simulink model "Test_iowahills_IIR"  (R2017b)
settings: Solver=FixedStepDiscrete  StartTime=0.0  StopTime=0.01  FixedStep=1/245.76e6  RelTol=1e-3  EnableMultiTasking=on
InitFcn:
  | Fs = 245.76e6;
  | Ts = 1 / Fs;
  | addpath('C:\Users\Keith\Documents\MATLAB\DigitalFilters\iowahills');
libraries: Library_SignalGeneration x2
settings Model: Creator=Keith  LastModifiedBy=Keith
settings OptimizationCC: BlockReduction=off  DefaultParameterBehavior=Inlined  BufferReuse=off  LifeSpan=inf
settings DebuggingCC: SFUnexpectedBacktrackingDiag=warning  SFNoUnconditionalDefaultTransitionDiag=warning  SFExecutionAtInitializationDiag=none
settings CodeAppCC: StateflowObjectComments=on
settings GRTTargetCC: TargetLangStandard=C89/C90 (ANSI)  GeneratePreprocessorConditionals=Disable all
settings ConfigComp: CovMetricSettings=dw  CovHtmlReporting=on  CovSaveCumulativeToWorkspaceVar=on  CovSaveSingleToWorkspaceVar=on  CovExternalEMLEnable=off

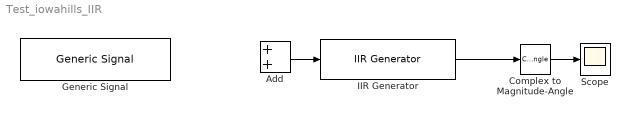
== system Test_iowahills_IIR ==
  Add : Sum
  Complex to Magnitude-Angle : ComplexToMagnitudeAngle  Output=Magnitude
  Generic Signal : Library_SignalGeneration/Generic Signal  fPoints=[0 245.76]*1e6  dPoints=[0 0]  tPoints=[0 0.01]  isPulsed=off  PRF=600e3  PD=.5e-6  FS=Fs
  IIR Generator : Library_SignalGeneration/IIR Generator  ihFilename=LPF_Shift.txt  shiftEnable=off  shiftFactor=0.5  bodeplt=0
      settings: AttributesFormatString=|
      | IIR File:  %<ihFilename>
      | Quad Shift: %<shiftEnable>,%<shiftFactor>
  Scope : Scope
  wires:
  IIR Generator/1 -> Complex to Magnitude-Angle/1
  Complex to Magnitude-Angle/1 -> Scope/1
  Add/1 -> IIR Generator/1
